simulink model "Ejemplosimulink"  (R2018b)
settings: Solver=FixedStepDiscrete  StartTime=0.0  StopTime=100  FixedStep=0.1  RelTol=1e-3  EnableMultiTasking=on
settings Model: Creator=jorge  LastModifiedBy=jorge
settings SolverCC: AutoInsertRateTranBlk=on
settings DataIOCC: LimitDataPoints=on
settings OptimizationCC: LifeSpan=inf
settings DebuggingCC: AllowSymbolicDim=off  SFUnexpectedBacktrackingDiag=warning  SFNoUnconditionalDefaultTransitionDiag=warning  SFExecutionAtInitializationDiag=none
settings SFSimCC: SimUseLocalCustomCode=off
settings RTWCC: RTWUseLocalCustomCode=off
settings CodeAppCC: StateflowObjectComments=on
settings GRTTargetCC: TargetLangStandard=C89/C90 (ANSI)  GeneratePreprocessorConditionals=Disable all
settings ConfigComp: CovMetricSettings=dw  CovHtmlReporting=on  CovSaveCumulativeToWorkspaceVar=on  CovSaveSingleToWorkspaceVar=on  CovShowResultsExplorer=off  CovExternalEMLEnable=off  CovSFcnEnable=off

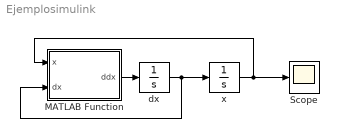
== system Ejemplosimulink ==
  MATLAB Function : MATLAB Function  TreatAsAtomicUnit=on
  Scope : Scope
  dx : Integrator
  x : Integrator  InitialCondition=0.5
  wires:
  MATLAB Function/1(ddx) -> dx/1
  dx/1 -> MATLAB Function/2(dx), x/1
  x/1 -> Scope/1, MATLAB Function/1(x)

== matlab function Ejemplosimulink/MATLAB Function ==
  data: x input; ddx output; dx input
function ddx = fcn(x,dx)
k = 0.01;
b = 0.001;
m = 0.5;
f = 0;
ddx= (1/m)*f-(b/m)*dx-(k/m)*x;
